simulink model "SimModel5"  (R2021a)
settings: Solver=FixedStepAuto  StartTime=0.0  StopTime=100  FixedStep=0.005  RelTol=1e-3
libraries: simulink x2, dspstat3 x1, pid_lib x1
settings Model: Creator=lucam  LastModifiedBy=lucam
settings SolverCC: ZeroCrossAlgorithm=Adaptive
settings DebuggingCC: IgnoredZcDiagnostic=none

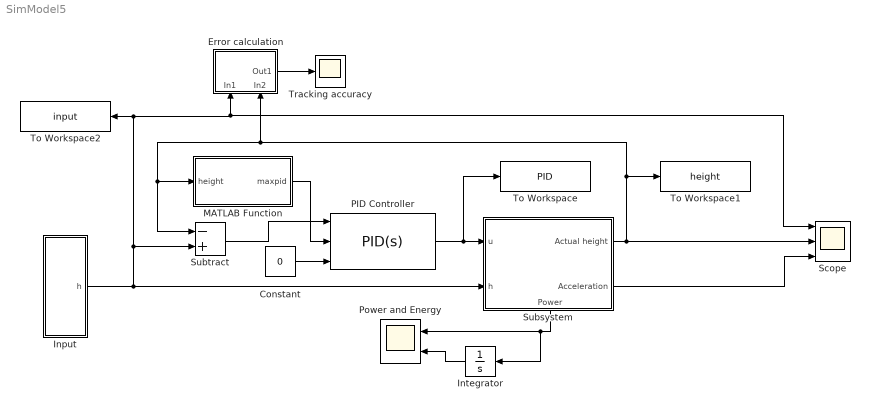
== system SimModel5 ==
  Constant : Constant  Value=0
  Error calculation : Subsystem
      settings: PortSchema="{\"entries\":[{\"content\":{\"sides\":[{\"content\":{\"connectorIds\":[\"In1\",\"In2\"]},\"type\":\"ConnectorPlacement.EquallySpacedRectSide\",\"uuid\":\"2e6f02a1-c3a7-4185-86c2-d40f93178419\"},{\"content\":{\"connectorIds\":[],\"side\":\"RIGHT\"},\"type\":\"ConnectorPlacement.EquallySpacedRectSide\",\"uuid\":\"00744759-e361-4441-9df3-2202444a8ed4\"},{\"content\":{\"connectorIds\":[],\"side\":\"TOP\"},\"type\":\"ConnectorPlacement.EquallySpacedRectSide\",\"uuid\":\"918a2cda-8d41-4eb5-91eb-c157fc3d1e5e\"},{\"content\":{\"connectorIds\":[\"Out1\"],\"side\":\"BOTTOM\"},\"type\":\"ConnectorPlacement.EquallySpacedRectSide\",\"uuid\":\"f3f3cf73-333a-4512-a63a-2dfc0e93eefb\"}]},\"type\":\"ConnectorPlacement.EquallySpacedConnector\",\"uuid\":\"7f411f1e-ef02-45d1-b6c2-c004038ded0e\"}],\"packageUris\":[\"http://schema.mathworks.com/mf0/Connector/R2020b\"],\"version\":\"1.0\"}"
  Input : Subsystem
  Integrator : Integrator
  MATLAB Function : MATLAB Function  TreatAsAtomicUnit=on
  PID Controller : pid_lib/PID Controller  Controller=PID  Form=Parallel  TimeDomain=Continuous-time  UseExternalTs=off  SampleTime=-1  IntegratorMethod=Forward Euler  FilterMethod=Forward Euler  ControllerParametersSource=internal  P=280  I=128  D=72  UseFilter=on  N=100  TunerSelectOption=Transfer Function Based (PID Tuner App)  InitialConditionSource=internal  InitialConditionForIntegrator=0  InitialConditionForFilter=0  DifferentiatorICPrevScaledInput=0  ExternalReset=none  TrackingMode=off  Kt=1  LimitOutput=on  SatLimitsSource=external  UpperSaturationLimit=100  LowerSaturationLimit=0  LinearizeAsGain=on  AntiWindupMode=clamping  Kb=1  POutMin=[]  POutMax=[]  IOutMin=[]  IOutMax=[]  DOutMin=[]  DOutMax=[]  NOutMin=[]  NOutMax=[]  SumOutMin=[]  SumOutMax=[]  SaturationOutMin=[]  SaturationOutMax=[]  PParamMin=[]  PParamMax=[]  IParamMin=[]  IParamMax=[]  DParamMin=[]  DParamMax=[]  NParamMin=[]  NParamMax=[]  KbParamMin=[]  KbParamMax=[]  KtParamMin=[]  KtParamMax=[]  KbOutMin=[]  KbOutMax=[]  KtOutMin=[]  KtOutMax=[]  IntegratorOutMin=[]  IntegratorOutMax=[]  FilterOutMin=[]  FilterOutMax=[]  SumI1OutMin=[]  SumI1OutMax=[]  SumI2OutMin=[]  SumI2OutMax=[]  SumI3OutMin=[]  SumI3OutMax=[]  SumI4OutMin=[]  SumI4OutMax=[]  SumDOutMin=[]  SumDOutMax=[]  DifferentiatorOutMin=[]  DifferentiatorOutMax=[]  FilterDiffOutCoefMin=[]  FilterDiffOutCoefMax=[]  ReciprocalOutMin=[]  ReciprocalOutMax=[]  SumDenOutMin=[]  SumDenOutMax=[]  SumNumOutMin=[]  SumNumOutMax=[]  DivideOutMin=[]  DivideOutMax=[]  UdiffTsProdOutMin=[]  UdiffTsProdOutMax=[]  NTsProdOutMin=[]  NTsProdOutMax=[]  UintegralTsProdOutMin=[]  UintegralTsProdOutMax=[]  UngainTsProdOutMin=[]  UngainTsProdOutMax=[]  IntegratorContinuousStateAttributes=''  IntegratorStateMustResolveToSignalObject=off  IntegratorRTWStateStorageClass=Auto  FilterContinuousStateAttributes=''  FilterStateMustResolveToSignalObject=off  FilterRTWStateStorageClass=Auto  ParallelPVariant=InternalParameters  IdealPVariant=Disabled  IVariant=InternalParameters  DVariant=InternalParameters  IntegratorVariant=Continuous  SatVariant=External  AWVariant=ContClampingParallel  PCopyVariant=Disabled  TRVariant=Disabled  FdbkBlocksVariant=Forward  IdealPFdbkVariant=Disabled  SatFdbkVariant=Disabled  DerivativeFilterVariant=ContFilter  NVariant=InternalParameters  NCopyVariant=Disabled  FilterICVariant=InternalICsFilter  IntegratorICVariant=InternalICs  ExternalResetVariant=Disabled  TRSumVariant=Passthrough  SumFdbkVariant=Disabled  SumVariant=Sum_PID  TsampFilterVariant=InternalTs  TsampNgainVariant=Passthrough  TsampIntegralVariant=Passthrough  ExternalSaturationOutDataTypeStr=Inherit: Same as second input
  Power and Energy : Scope  NumInputPorts=2
  Scope : Scope  NumInputPorts=3
  Subsystem : Subsystem
      settings: PortSchema="{\"entries\":[{\"content\":{\"sides\":[{\"content\":{\"connectorIds\":[\"In1\",\"In2\"]},\"type\":\"ConnectorPlacement.EquallySpacedRectSide\",\"uuid\":\"572f826c-3722-4f31-aa09-a23c7543edd6\"},{\"content\":{\"connectorIds\":[\"Out1\",\"Out2\"],\"side\":\"RIGHT\"},\"type\":\"ConnectorPlacement.EquallySpacedRectSide\",\"uuid\":\"1fb53aaa-4365-43d4-913e-268d0517c7d9\"},{\"content\":{\"connectorIds\":[],\"side\":\"TOP\"},\"type\":\"ConnectorPlacement.EquallySpacedRectSide\",\"uuid\":\"2d6f6f11-5226-4b68-83e8-9a360e280de8\"},{\"content\":{\"connectorIds\":[\"Out3\"],\"side\":\"BOTTOM\"},\"type\":\"ConnectorPlacement.EquallySpacedRectSide\",\"uuid\":\"574730be-9116-496a-aef5-d7f71710a288\"}]},\"type\":\"ConnectorPlacement.EquallySpacedConnector\",\"uuid\":\"fba5509b-faba-4204-acbc-ad4d250f8daa\"}],\"packageUris\":[\"http://schema.mathworks.com/mf0/Connector/R2020b\"],\"version\":\"1.0\"}"
  Subtract : Sum  Inputs=-+
  To Workspace : ToWorkspace  VariableName=PID  SaveFormat=Timeseries  SampleTime=-1
  To Workspace1 : ToWorkspace  VariableName=height  SaveFormat=Timeseries  SampleTime=-1
  To Workspace2 : ToWorkspace  VariableName=input  SaveFormat=Timeseries  SampleTime=-1
  Tracking accuracy : Scope
  wires:
  Input/1(h) -> Scope/1, Error calculation/1(In1), To Workspace2/1, Subtract/2, Subsystem/2(h)
  Integrator/1 -> Power and Energy/2
  Error calculation/1(Out1) -> Tracking accuracy/1
  Subtract/1 -> PID Controller/1
  Subsystem/1(Actual height) -> MATLAB Function/1(height), Subtract/1, Error calculation/2(In2), To Workspace1/1, Scope/2
  Subsystem/3(Power) -> Integrator/1, Power and Energy/1
  PID Controller/1 -> To Workspace/1, Subsystem/1(u)
  MATLAB Function/1(maxpid) -> PID Controller/2
  Subsystem/2(Acceleration) -> Scope/3
  Constant/1 -> PID Controller/3

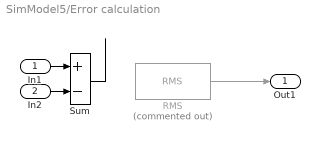
== system SimModel5/Error calculation ==
  In1 : Inport
  In2 : Inport  Port=2
  RMS : dspstat3/RMS  Commented=on  run=on  directionMode=Each column  dimension=1  reset_popup=None
  Sum : Sum  Inputs=+-
  Out1 : Outport
  wires:
  In1/1 -> Sum/1
  In2/1 -> Sum/2
  RMS/1 -> Out1/1
  Sum/1 -> ?

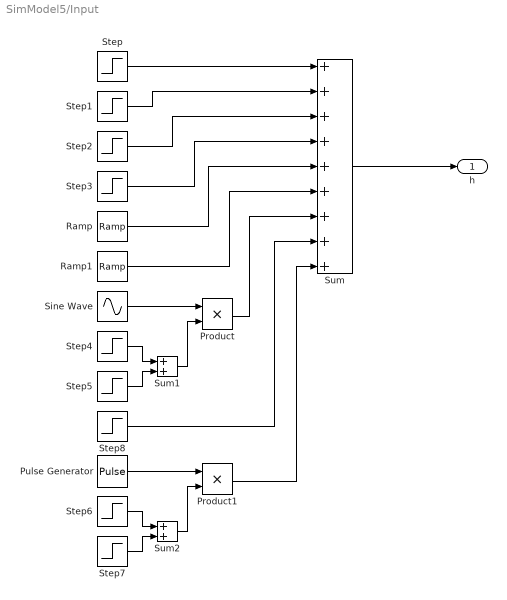
== system SimModel5/Input ==
  Product : Product
  Product1 : Product
  Pulse Generator : DiscretePulseGenerator  PulseType=Time based  PulseWidth=50
  Ramp : simulink/Sources/Ramp  slope=0.05  start=40  InitialOutput=0
  Ramp1 : simulink/Sources/Ramp  slope=-0.05  start=50  InitialOutput=0
  Sine Wave : Sin  Amplitude=0.3  SampleTime=0
  Step : Step  Time=0  After=1.44  SampleTime=0
  Step1 : Step  Time=10  After=-1.44  SampleTime=0
  Step2 : Step  Time=20  After=0.4  SampleTime=0
  Step3 : Step  Time=30  After=-0.4  SampleTime=0
  Step4 : Step  Time=60  SampleTime=0
  Step5 : Step  Time=70  After=-1  SampleTime=0
  Step6 : Step  Time=80  SampleTime=0
  Step7 : Step  Time=90  After=-1  SampleTime=0
  Step8 : Step  Time=80  After=-0.3  SampleTime=0
  Sum : Sum  Inputs=+++++++++
  Sum1 : Sum
  Sum2 : Sum
  h : Outport
  wires:
  Step1/1 -> Sum/2
  Step3/1 -> Sum/4
  Step/1 -> Sum/1
  Step2/1 -> Sum/3
  Step4/1 -> Sum1/1
  Sine Wave/1 -> Product/1
  Step5/1 -> Sum1/2
  Sum1/1 -> Product/2
  Ramp/1 -> Sum/5
  Ramp1/1 -> Sum/6
  Product/1 -> Sum/7
  Step6/1 -> Sum2/1
  Sum2/1 -> Product1/2
  Pulse Generator/1 -> Product1/1
  Step7/1 -> Sum2/2
  Product1/1 -> Sum/9
  Step8/1 -> Sum/8
  Sum/1 -> h/1

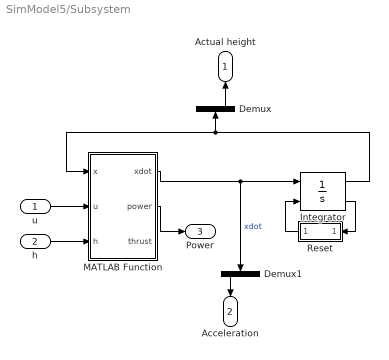
== system SimModel5/Subsystem ==
  u : Inport
  h : Inport  Port=2
  Demux : Demux  Outputs=2
  Demux1 : Demux  Outputs=2
  Integrator : Integrator  ExternalReset=rising  InitialCondition=[0;0]  LimitOutput=on  UpperSaturationLimit=[inf,1.44]  LowerSaturationLimit=[-inf,0]  ShowSaturationPort=on  ZeroCross=off
  MATLAB Function : MATLAB Function  TreatAsAtomicUnit=on
  Reset : Subsystem
  Actual height : Outport
  Acceleration : Outport  Port=2
  Power : Outport  Port=3
  wires:
  Integrator/1 -> MATLAB Function/1(x), Demux/1
  MATLAB Function/2(power) -> Power/1
  Integrator/2 -> Reset/1(In1)
  MATLAB Function/1(xdot) -> Integrator/1, Demux1/1  "xdot"
  h/1 -> MATLAB Function/3(h)
  Reset/1(Out1) -> Integrator/2
  Demux/2 -> Actual height/1
  u/1 -> MATLAB Function/2(u)
  Demux1/1 -> Acceleration/1

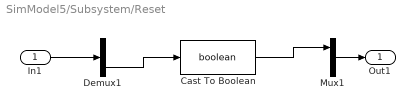
== system SimModel5/Subsystem/Reset ==
  In1 : Inport
  Cast To Boolean : DataTypeConversion  OutDataTypeStr=boolean
  Demux1 : Demux  Outputs=2
  Mux1 : Mux  Inputs=2
  Out1 : Outport
  wires:
  Cast To Boolean/1 -> Mux1/1
  Demux1/2 -> Cast To Boolean/1
  Mux1/1 -> Out1/1
  In1/1 -> Demux1/1

== matlab function SimModel5/MATLAB Function ==
  data: height input; maxpid output
function maxpid = maxpid(height)

cartmass        = 0.454;      %kg
armmass         = 0.04;        %kg
cablemass       = 2*(0.462*0.190*height+0.335*0.190); %kg

mass = cartmass + armmass + cablemass; %kg

maxt = mass * 9.81 -0.5;

maxpid = 0.000106460047187 * maxt^6 + 0.001682145469029 * maxt^5 - 0.085966748628573 * maxt^4 + 0.915086428052733 * maxt^3 - 4.301170611461207 * maxt^2 + 19.048979026808645 * maxt - 0.819624990299465;

== matlab function SimModel5/Subsystem/MATLAB Function ==
  data: x input; u input; xdot output; h input; power output; thrust output
function [xdot,power,thrust] = model(x,u,h)
%inputs - x: (2x1) state vector
%         x(1)- v   m/s
%         x(2)- z   m
%       - u:  control vector
%         u(1)- engine throttle as percentage

g=9.81;

cartmass        = 0.454;      %kg
armmass         = 0.04;        %kg
mukin           = 0.14;
mustatic        = 0.17;
normalforce     = 7.5;        %N  
cablemass       = 2*(0.462*0.190*x(2)+0.335*0.190); %kg

m = cartmass + armmass + cablemass; %kg
thrust=2*(-1.406748142176356e-10*u^6+3.062978540873029e-08*u^5-2.097995902290989e-06*u^4+3.239235806681329e-05*u^3+0.001982324981180*u^2+0.021260289345294*u+0.164761238254325);
power=2*(-7.965663601959184e-09*u^6 +1.901136049289777e-06*u^5 -1.589619337574908e-04*u^4 +0.005425679690860*u^3 -0.030524707578218*u^2 +0.794872021052043*u +2.959442083749500);
staticfriction = sign(h-x(2)) * mustatic * normalforce;
dynamicfriction = sign(x(1)) * mukin * normalforce;

A=[1/m,0;0,1];

if (x(2)>=1.44&&h>=1.44)||(x(2)<=0&&h<=0)
    xdot=[0;0];
else
    if x(1)==0
        xdot=A*[thrust-m*g-staticfriction;x(1)];
    else
        xdot=A*[thrust-m*g-dynamicfriction;x(1)];
    end
end
